simulink model "SD2231_Lab1_2024_PIDController"  (R2023a)
settings: Solver=FixedStepAuto  StartTime=0.0  StopTime=inf  FixedStep=0.001  RelTol=1e-3  EnableMultiTasking=on
values from neighbouring files (symbols this model uses):
  K_brake = K_brake(3)    [initial_student.m]    (also in initial_student_final.m)
  K_em = K_em(3)    [initial_student.m]    (also in initial_student_final.m)
undefined symbols (not defined in the file or in its folder): DiscIntNeverNeededParam, Veh
libraries: CarMaker4SL x37, SignalEditorBlockLib x2, autolibmappedmotor x2
(part 1 of 3)
settings Model: ExtModeTrigMode=oneshot  Creator=cs  LastModifiedBy=Student
settings SolverCC: AlgebraicLoopSolver=TrustRegion
settings DataIOCC: SaveFormat=Array  SignalLoggingSaveFormat=ModelDataLogs  ReturnWorkspaceOutputs=off  SignalLoggingName=sigsOut
settings OptimizationCC: BooleanDataType=off  OptimizeBlockIOStorage=off  BufferReuse=off  GlobalBufferReuse=off  ExpressionFolding=off  ExpressionDepthLimit=2147483647  LocalBlockOutputs=off  InitFltsAndDblsToZero=on  LifeSpan=inf  OptimizeDataStoreBuffers=off  BusAssignmentInplaceUpdate=off
settings DebuggingCC: SaveWithParameterizedLinksMsg=none  UnderspecifiedInitializationDetection=Classic  MergeDetectMultiDrivingBlocksExec=none  SignalResolutionControl=TryResolveAllWithWarning  MultiTaskDSMMsg=warning  MultiTaskCondExecSysMsg=none  FcnCallInpInsideContextMsg=warning  UnconnectedInputMsg=warning  UnconnectedOutputMsg=warning  UnconnectedLineMsg=warning  StateNameClashWarn=warning  SFUnexpectedBacktrackingDiag=warning  SFNoUnconditionalDefaultTransitionDiag=warning  ArithmeticOperatorsInVariantConditions=warning
settings HardwareCC: ProdBitPerPointer=32  ProdBitPerSizeT=32  ProdBitPerPtrDiffT=32  ProdLargestAtomicFloat=None  ProdIntDivRoundTo=Undefined  ProdEndianess=Unspecified  ProdWordSize=32  ProdHWDeviceType=32-bit Generic  TargetUnknown=on
settings ModelReferenceCC: EnableRefExpFcnMdlSchedulingChecks=on  PropagateSignalLabelsOutOfModel=off
settings SFSimCC: SimUseLocalCustomCode=off  CustomCodeUndefinedFunction=UseInterfaceOnly
settings RTWCC: SystemTargetFile=grt_malloc.tlc  TemplateMakefile=grt_malloc_default_tmf  RTWUseLocalCustomCode=off
settings CodeAppCC: MaxIdLength=63  StateflowObjectComments=on
settings GRTTargetCC: TargetFcnLib=ansi_tfl_tmw.mat  TargetLangStandard=C89/C90 (ANSI)  CombineOutputUpdateFcns=off  GRTInterface=on  UseMalloc=on  ExtModeMexFile=noextcomm
settings ConfigComp: CovMetricSettings=dw  CovSaveCumulativeToWorkspaceVar=on  CovSaveSingleToWorkspaceVar=on  CovExternalEMLEnable=off

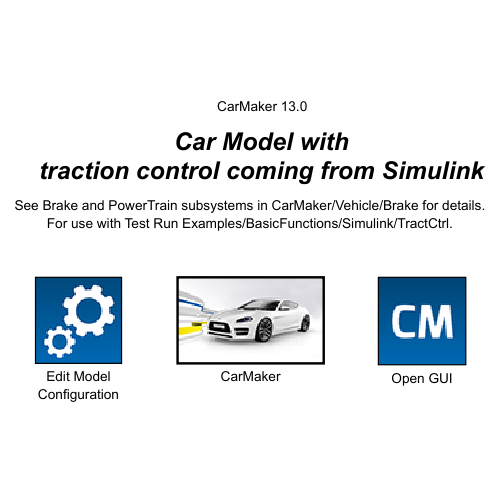
[thumbnail: Simulink's stored preview of the top-level diagram]
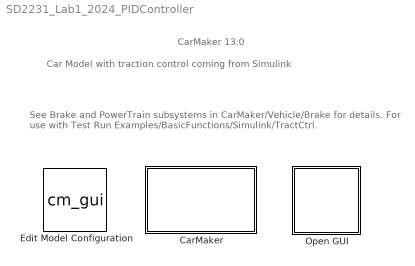
== system SD2231_Lab1_2024_PIDController ==
  note: Car Model with
      | traction control coming from Simulink
  note: See Brake and PowerTrain subsystems in CarMaker/Vehicle/Brake for details.
      | For use with Test Run Examples/BasicFunctions/Simulink/TractCtrl.
  note: CarMaker 13.0
  CarMaker : Subsystem  TreatAsAtomicUnit=on
      mask Display: image(imread('CarMakerSys.png'));
  Edit Model Configuration : S-Function  FunctionName=cm_gui  SFunctionDeploymentMode=off  EnableBusSupport=off
      settings: OpenFcn=cmmodelconf('edit');
      mask Display: image(imread('ModelConfig.png'));
  Open GUI : Subsystem  LoadFcn=if ~length(which('cmself')), cmenv; end
      settings: OpenFcn=cmblockmagic('gui_fix_display'); CM_Simulink
      mask Display: image(imread('CarMakerGUI.png'));

== system SD2231_Lab1_2024_PIDController/CarMaker ==
  Bus Creator : BusCreator  Inputs=6
  CM_FIRST : Subsystem
  CM_LAST : Subsystem
  CarMaker data : Subsystem
  DrivMan : Subsystem
  Ground : Ground
  IPG Vehicle : Subsystem
  Road friction : Subsystem
  Terminator : Terminator
  VehicleControl : Subsystem
  Your ABS Controller : Subsystem
  Your Traction Controller : Subsystem
  Your observer : Subsystem
  Your tyre force mapping : Subsystem
  wires:
  VehicleControl/2(Vhcl.Model.Source) -> IPG Vehicle/2(Vhcl.Model.Source)
  VehicleControl/7(VhclCtrl.PT) -> IPG Vehicle/7(VhclCtrl.PT)
  VehicleControl/6(VhclCtrl.Brake) -> IPG Vehicle/6(VhclCtrl.Brake)
  VehicleControl/5(Vhcl.Misc) -> IPG Vehicle/5(Vhcl.Misc)
  VehicleControl/4(Vhcl.Wheel.In) -> IPG Vehicle/4(Vhcl.Wheel.In)
  VehicleControl/3(VhclCtrl.Steering) -> IPG Vehicle/3(VhclCtrl.Steering)
  VehicleControl/1(Sync_Out) -> IPG Vehicle/1(Sync_In)
  IPG Vehicle/1(Sync_Out) -> CM_LAST/1(Sync_In)
  Ground/1 -> CM_FIRST/1(Sync_In)
  CM_LAST/1(Sync_Out) -> Terminator/1
  CM_FIRST/1(Sync_Out) -> DrivMan/1(Sync_In)
  CM_FIRST/2(Env.Misc) -> DrivMan/2(Env.Misc)
  DrivMan/1(Sync_Out) -> VehicleControl/1(Sync_In)
  DrivMan/2(DrivMan.Out) -> VehicleControl/2(DrivMan.In)
  Your ABS Controller/4(RRBrakeAdjust) -> Bus Creator/6
  Your observer/1(CarMaker bus data out) -> Your Traction Controller/1(CarMaker bus data), Your ABS Controller/1(CarMaker bus data)
  Your Traction Controller/2(RR TrqReqSignal (0-1)) -> Bus Creator/2
  Bus Creator/1 -> IPG Vehicle/8(SD2231.data)
  Your ABS Controller/2(FRBrakeAdjust) -> Bus Creator/4
  Your ABS Controller/1(FLBrakeAdjust) -> Bus Creator/3
  Your ABS Controller/3(RLBrakeAdjust) -> Bus Creator/5
  CarMaker data/1(CarMaker bus data) -> Your observer/1(CarMaker bus data)
  Your observer/2(Tyre slip bus data out) -> Your Traction Controller/2(Tyre slip bus data), Your tyre force mapping/1(Tyre slip bus data out), Your ABS Controller/2(Tyre slip bus data)
  Your Traction Controller/1(LR TrqReqSignal (0-1)) -> Bus Creator/1

== system SD2231_Lab1_2024_PIDController/Open GUI ==
  S-Function : S-Function  FunctionName=cm_gui  SFunctionDeploymentMode=off  EnableBusSupport=off

== system SD2231_Lab1_2024_PIDController/CarMaker/CM_FIRST ==
  Sync_In : Inport
  BusCreator1 : BusCreator  Inputs=8
  BusCreator2 : BusCreator  Inputs=6
  Demux1 : Demux  Outputs=14
      settings: DisplayOption=none
  Environment : S-Function  FunctionName=CM_Sfun  Parameters='Environment'  SFunctionDeploymentMode=off  EnableBusSupport=off
  IoIn : S-Function  FunctionName=CM_Sfun  Parameters='IoIn'  SFunctionDeploymentMode=off  EnableBusSupport=off
  Terminator : Terminator
  Sync_Out : Outport  VectorParamsAs1DForOutWhenUnconnected=off
  Env.Misc : Outport  Port=2  VectorParamsAs1DForOutWhenUnconnected=off
  wires:
  BusCreator2/1 -> Terminator/1  "IF Environment (in)"
  BusCreator1/1 -> Env.Misc/1
  Demux1/14 -> BusCreator2/6  "Env sRoad"
  Demux1/13 -> BusCreator2/5  "Env PoI_GCS Elev"
  Demux1/12 -> BusCreator2/4  "Env PoI_GCS Lat"
  Demux1/11 -> BusCreator2/3  "Env PoI_GCS Long"
  Demux1/10 -> BusCreator2/2  "Env Time"
  Demux1/9 -> BusCreator2/1  "Env yDay"
  Demux1/8 -> BusCreator1/8  "Env WindVel_tot z"
  Demux1/7 -> BusCreator1/7  "Env WindVel_tot y"
  Demux1/6 -> BusCreator1/6  "Env WindVel_tot x"
  Demux1/5 -> BusCreator1/5  "Env SolarRadiation"
  Demux1/4 -> BusCreator1/4  "Env AirHumidity"
  Demux1/3 -> BusCreator1/3  "Env AirPressure"
  Demux1/2 -> BusCreator1/2  "Env AirDensity"
  Demux1/1 -> BusCreator1/1  "Env Temperature"
  Environment/2 -> Demux1/1
  Environment/1 -> Sync_Out/1
  IoIn/1 -> Environment/1
  Sync_In/1 -> IoIn/1

== system SD2231_Lab1_2024_PIDController/CarMaker/CM_LAST ==
  Sync_In : Inport
  CM_User : S-Function  FunctionName=CM_Sfun  Parameters='CM_User'  SFunctionDeploymentMode=off  EnableBusSupport=off
  IoOut : S-Function  FunctionName=CM_Sfun  Parameters='IoOut'  SFunctionDeploymentMode=off  EnableBusSupport=off
  Sync_Out : Outport  VectorParamsAs1DForOutWhenUnconnected=off
  wires:
  IoOut/1 -> Sync_Out/1
  CM_User/1 -> IoOut/1
  Sync_In/1 -> CM_User/1

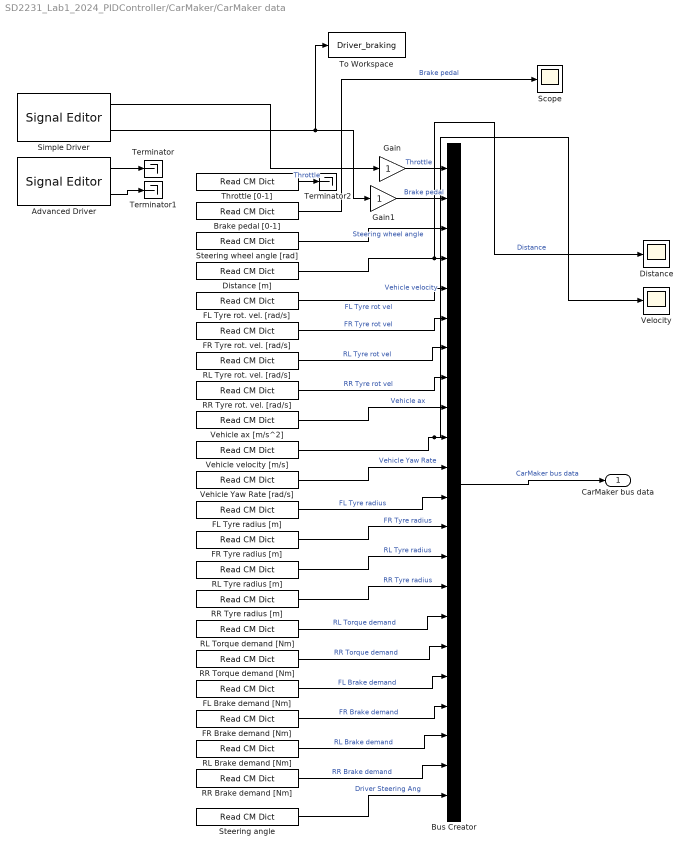
== system SD2231_Lab1_2024_PIDController/CarMaker/CarMaker data ==
  Advanced Driver : SignalEditorBlockLib/Signal Editor  FileName=DriverGas_Advanced.mat  ActiveScenario=Scenario  ActiveSignal=Brake  IsBus=off  OutputBusObjectStr=Bus: BusObject  SampleTime=0  ZeroCross=off  OutputAfterFinalValue=Holding final value  Unit=inherit  PreserveSignalName=on  ApplySigPropsToAllScenarios=off
  Brake pedal [0-1] : CarMaker4SL/Read CM Dict  xname=Driver.Brake  xsync=off  xstime=Continuous
  Bus Creator : BusCreator  Inputs=22
  Distance : Scope
  Distance [m] : CarMaker4SL/Read CM Dict  xname=Vhcl.Distance  xsync=off  xstime=Continuous
  FL Brake demand [Nm] : CarMaker4SL/Read CM Dict  xname=Vhcl.FL.Trq_Brake  xsync=off  xstime=Continuous
  FL Tyre radius [m] : CarMaker4SL/Read CM Dict  xname=Car.WFL.Radius  xsync=off  xstime=Continuous
  FL Tyre rot. vel. [rad/s] : CarMaker4SL/Read CM Dict  xname=Car.WheelSpd_FL  xsync=off  xstime=Continuous
  FR Brake demand [Nm] : CarMaker4SL/Read CM Dict  xname=Vhcl.FR.Trq_Brake  xsync=off  xstime=Continuous
  FR Tyre radius [m] : CarMaker4SL/Read CM Dict  xname=Car.WFR.Radius  xsync=off  xstime=Continuous
  FR Tyre rot. vel. [rad/s] : CarMaker4SL/Read CM Dict  xname=Car.WheelSpd_FR  xsync=off  xstime=Continuous
  Gain : Gain
  Gain1 : Gain
  RL Brake demand [Nm] : CarMaker4SL/Read CM Dict  xname=Vhcl.RL.Trq_Brake  xsync=off  xstime=Continuous
  RL Torque demand [Nm] : CarMaker4SL/Read CM Dict  xname=Vhcl.RL.Trq_T2W  xsync=off  xstime=Continuous
  RL Tyre radius [m] : CarMaker4SL/Read CM Dict  xname=Car.WRL.Radius  xsync=off  xstime=Continuous
  RL Tyre rot. vel. [rad/s] : CarMaker4SL/Read CM Dict  xname=Car.WheelSpd_RL  xsync=off  xstime=Continuous
  RR Brake demand [Nm] : CarMaker4SL/Read CM Dict  xname=Vhcl.RR.Trq_Brake  xsync=off  xstime=Continuous
  RR Torque demand [Nm] : CarMaker4SL/Read CM Dict  xname=Vhcl.RR.Trq_T2W  xsync=off  xstime=Continuous
  RR Tyre radius [m] : CarMaker4SL/Read CM Dict  xname=Car.WRR.Radius  xsync=off  xstime=Continuous
  RR Tyre rot. vel. [rad/s] : CarMaker4SL/Read CM Dict  xname=Car.WheelSpd_RR  xsync=off  xstime=Continuous
  Scope : Scope
  Simple Driver : SignalEditorBlockLib/Signal Editor  FileName=DriverGas.mat  ActiveScenario=Scenario  ActiveSignal=Brake  IsBus=off  OutputBusObjectStr=Bus: BusObject  SampleTime=0  ZeroCross=off  OutputAfterFinalValue=Holding final value  Unit=inherit  PreserveSignalName=on  ApplySigPropsToAllScenarios=off
  Steering angle : CarMaker4SL/Read CM Dict  xname=Driver.Steer.Ang  xsync=off  xstime=Continuous
  Steering wheel angle [rad] : CarMaker4SL/Read CM Dict  xname=Driver.Steer.Ang  xsync=off  xstime=Continuous
  Terminator : Terminator
  Terminator1 : Terminator
  Terminator2 : Terminator
  Throttle [0-1] : CarMaker4SL/Read CM Dict  xname=Driver.Gas  xsync=off  xstime=Continuous
  To Workspace : ToWorkspace  VariableName=Driver_braking  SaveFormat=Timeseries  SampleTime=-1
  Vehicle Yaw Rate [rad/s] : CarMaker4SL/Read CM Dict  xname=Car.YawRate  xsync=off  xstime=Continuous
  Vehicle ax [m/s^2] : CarMaker4SL/Read CM Dict  xname=Car.ax  xsync=off  xstime=Continuous
  Vehicle velocity [m/s] : CarMaker4SL/Read CM Dict  xname=Car.v  xsync=off  xstime=Continuous
  Velocity : Scope
  CarMaker bus data : Outport  VectorParamsAs1DForOutWhenUnconnected=off
  wires:
  RR Tyre rot. vel. [rad/s]/1 -> Bus Creator/8  "RR Tyre rot vel"
  RL Tyre rot. vel. [rad/s]/1 -> Bus Creator/7  "RL Tyre rot vel"
  Distance [m]/1 -> Distance/1, Bus Creator/4  "Distance"
  FR Tyre rot. vel. [rad/s]/1 -> Bus Creator/6  "FR Tyre rot vel"
  Brake pedal [0-1]/1 -> Scope/1  "Brake pedal"
  Vehicle ax [m/s^2]/1 -> Bus Creator/9  "Vehicle ax"
  Steering wheel angle [rad]/1 -> Bus Creator/3  "Steering wheel angle"
  Throttle [0-1]/1 -> Terminator2/1  "Throttle"
  Vehicle velocity [m/s]/1 -> Velocity/1, Bus Creator/10  "Vehicle velocity"
  FL Tyre rot. vel. [rad/s]/1 -> Bus Creator/5  "FL Tyre rot vel"
  Vehicle Yaw Rate [rad/s]/1 -> Bus Creator/11  "Vehicle Yaw Rate"
  FL Tyre radius [m]/1 -> Bus Creator/12  "FL Tyre radius"
  FR Tyre radius [m]/1 -> Bus Creator/13  "FR Tyre radius"
  RL Tyre radius [m]/1 -> Bus Creator/14  "RL Tyre radius"
  RR Tyre radius [m]/1 -> Bus Creator/15  "RR Tyre radius"
  Bus Creator/1 -> CarMaker bus data/1  "CarMaker bus data"
  RL Torque demand [Nm]/1 -> Bus Creator/16  "RL Torque demand"
  RR Torque demand [Nm]/1 -> Bus Creator/17  "RR Torque demand"
  FL Brake demand [Nm]/1 -> Bus Creator/18  "FL Brake demand"
  FR Brake demand [Nm]/1 -> Bus Creator/19  "FR Brake demand"
  RL Brake demand [Nm]/1 -> Bus Creator/20  "RL Brake demand"
  RR Brake demand [Nm]/1 -> Bus Creator/21  "RR Brake demand"
  Gain/1 -> Bus Creator/1  "Throttle"
  Gain1/1 -> Bus Creator/2  "Brake pedal"
  Steering angle/1 -> Bus Creator/22  "Driver Steering Ang"
  Simple Driver/1 -> Gain/1
  Advanced Driver/1 -> Terminator/1
  Simple Driver/2 -> To Workspace/1, Gain1/1
  Advanced Driver/2 -> Terminator1/1

== system SD2231_Lab1_2024_PIDController/CarMaker/DrivMan ==
  note: There's rarely a reason to override DrivMan signals.
      | Use the VehicleControl interface for this purpose.
  Sync_In : Inport
  Env.Misc : Inport  Port=2
  BusCreator : BusCreator  Inputs=20
  Demux : Demux  Outputs=20
      settings: DisplayOption=none
  DrivMan : S-Function  FunctionName=CM_Sfun  Parameters='DrivMan'  SFunctionDeploymentMode=off  EnableBusSupport=off
  Sync_Out : Outport  VectorParamsAs1DForOutWhenUnconnected=off
  DrivMan.Out : Outport  Port=2  VectorParamsAs1DForOutWhenUnconnected=off
  wires:
  Demux/8 -> BusCreator/8  "DrivMan SelectorCtrl"
  Demux/7 -> BusCreator/7  "DrivMan UserSignal4"
  Demux/6 -> BusCreator/6  "DrivMan UserSignal3"
  Demux/5 -> BusCreator/5  "DrivMan UserSignal2"
  Demux/4 -> BusCreator/4  "DrivMan UserSignal1"
  Demux/3 -> BusCreator/3  "DrivMan UserSignal0"
  Demux/2 -> BusCreator/2  "DrivMan Key"
  Demux/1 -> BusCreator/1  "DrivMan SST"
  Env.Misc/1 -> DrivMan/2
  Sync_In/1 -> DrivMan/1
  DrivMan/1 -> Sync_Out/1
  BusCreator/1 -> DrivMan.Out/1
  DrivMan/2 -> Demux/1
  Demux/9 -> BusCreator/9  "DrivMan DigitalSelectorCtrl0"
  Demux/10 -> BusCreator/10  "DrivMan DigitalSelectorCtrl1"
  Demux/11 -> BusCreator/11  "DrivMan DigitalSelectorCtrl2"
  Demux/20 -> BusCreator/20  "DrivMan Steering Trq"
  Demux/19 -> BusCreator/19  "DrivMan Steering AngAcc"
  Demux/18 -> BusCreator/18  "DrivMan Steering AngVel"
  Demux/17 -> BusCreator/17  "DrivMan Steering Ang"
  Demux/16 -> BusCreator/16  "DrivMan Gas"
  Demux/15 -> BusCreator/15  "DrivMan Clutch"
  Demux/14 -> BusCreator/14  "DrivMan BrakePark"
  Demux/13 -> BusCreator/13  "DrivMan Brake"
  Demux/12 -> BusCreator/12  "DrivMan GearNo"

== system SD2231_Lab1_2024_PIDController/CarMaker/IPG Vehicle ==
  Sync_In : Inport
  Vhcl.Model.Source : Inport  Port=2
  VhclCtrl.Steering : Inport  Port=3
  Vhcl.Wheel.In : Inport  Port=4
  Vhcl.Misc : Inport  Port=5
  VhclCtrl.Brake : Inport  Port=6
  VhclCtrl.PT : Inport  Port=7
  SD2231.data : Inport  Port=8
  Brake : Subsystem
  CarAndTrailer : Subsystem
  PowerTrain : Subsystem
  Stop Simulation : Stop
  VehicleSource_BuiltIn : Subsystem  mask(Compare To Constant){relop=~=, const=1, OutDataTypeStr=boolean, ZeroCross=off}
      mask prompts: relop "Simulink:masks:Operator_MP"; const "Simulink:masks:ConstantValue_MP"; OutDataTypeStr "Simulink:masks:OutputDataType_MP"; ZeroCross "Simulink:masks:EnableZerocrossingDetection_MP"
      mask help: Simulink:masks:CompareToConstant_MD
      mask init:
      | blkName = gcb;
      | 
      | if strcmp(get_param(gcbh,'OutDataTypeStr'),'boolean')
      | 	setValue = 'boolean';
      | else
      | 	setValue = 'fixdt(0, 8)';
      | end
      | 
      | set_param([blkName,'/Compare'],'relop',relop, ...
      | 	'OutDataTypeStr', setValue, 'ZeroCross', ZeroCross);
      | 
      | str = [relop,' C']; %default
      | 
      | const_str = get_param(blkName, 'const');
      | 
      | if isempty(strfind(const_str, ' ')) && isempty(strfind(const_str, ','))
      |     % scalar or single expression
      |     if isempty(str2num(const_str))
      |         %expression
      |         str = [relop, ' ', const_str];
      |     elseif length(const) == 1
      |         str = [relop,' ',num2str(double(const))];
      |     end
      | end
      mask TypeOptions relop: == | ~= | < | <= | >= | >
      mask TypeOptions OutDataTypeStr: Simulink:masks:uint8 | Simulink:masks:boolean
      mask Callback ZeroCross: sl('zeroCrossEnable', gcbh);
      mask Display: disp(str)
  Sync_Out : Outport  VectorParamsAs1DForOutWhenUnconnected=off
  wires:
  VhclCtrl.PT/1 -> PowerTrain/3(VhclCtrl.PT)
  Brake/1(Sync_Out) -> PowerTrain/1(Sync_In)
  CarAndTrailer/1(Sync_Out) -> Brake/1(Sync_In)
  CarAndTrailer/2(Brake.IF.In) -> Brake/2(Brake.IF.In)
  VhclCtrl.Brake/1 -> Brake/3(VhclCtrl.Brake)
  PowerTrain/1(Sync_Out) -> Sync_Out/1
  Vhcl.Misc/1 -> CarAndTrailer/4(Vhcl.Misc)
  Vhcl.Wheel.In/1 -> CarAndTrailer/3(Vhcl.Wheel.In)
  VhclCtrl.Steering/1 -> CarAndTrailer/2(VhclCtrl.Steering)
  Sync_In/1 -> CarAndTrailer/1(Sync_In)
  Vhcl.Model.Source/1 -> VehicleSource_BuiltIn/1(u)
  VehicleSource_BuiltIn/1(y) -> Stop Simulation/1
  Brake/2(Vhcl.Wheel.PT) -> PowerTrain/2(Vhcl.Wheel.PT)
  SD2231.data/1 -> PowerTrain/6(SD2232.data), Brake/4(SD2231.Data)
  CarAndTrailer/3(Car.Trq_T2W) -> PowerTrain/5(Car.TrqT2W)
  Brake/3(Brake.IF.Out) -> PowerTrain/4(Brake.IF.Out)

== system SD2231_Lab1_2024_PIDController/CarMaker/Road friction ==
  Constant : Constant  Value=Veh.mu
  Write CM Dict : CarMaker4SL/Write CM Dict  xname=Car.muRoadFL  xsync=off
  Write CM Dict1 : CarMaker4SL/Write CM Dict  xname=Car.muRoadFR  xsync=off
  Write CM Dict2 : CarMaker4SL/Write CM Dict  xname=Car.muRoadRL  xsync=off
  Write CM Dict3 : CarMaker4SL/Write CM Dict  xname=Car.muRoadRR  xsync=off
  wires:
  Constant/1 -> Write CM Dict1/1, Write CM Dict/1, Write CM Dict3/1, Write CM Dict2/1

== system SD2231_Lab1_2024_PIDController/CarMaker/VehicleControl ==
  note: <Your model here>
  note: When implementing a vehicle control model,
      | be sure to add '-disablevehiclecontrol' to the command line arguments
      | in the CarMaker Model Configuration block.
      | Otherwise your model will possibly not see the original DrivMan signals
      | on its inputs, but those of a currently activated C-coded vehicle control model instead.
  Sync_In : Inport
  DrivMan.In : Inport  Port=2
  Bus Creator2 : BusCreator  Inputs=2
  CreateBus Vhcl.Misc : Subsystem
  CreateBus Vhcl.Wheel.In : Subsystem
  CreateBus VhclCtrl : Subsystem
  CreateBus VhclCtrl.PT : Subsystem
  CreateBus VhclCtrl.Steering : Subsystem
  Demux2 : Demux  Outputs=2
      settings: DisplayOption=none
  VehicleControl : S-Function  FunctionName=CM_Sfun  Parameters='VehicleControl'  SFunctionDeploymentMode=off  EnableBusSupport=off
  VehicleControlUpd : S-Function  FunctionName=CM_Sfun  Parameters='VehicleControlUpd'  SFunctionDeploymentMode=off  EnableBusSupport=off
  Sync_Out : Outport  VectorParamsAs1DForOutWhenUnconnected=off
  Vhcl.Model.Source : Outport  Port=2  VectorParamsAs1DForOutWhenUnconnected=off
  VhclCtrl.Steering : Outport  Port=3  VectorParamsAs1DForOutWhenUnconnected=off
  Vhcl.Wheel.In : Outport  Port=4  VectorParamsAs1DForOutWhenUnconnected=off
  Vhcl.Misc : Outport  Port=5  VectorParamsAs1DForOutWhenUnconnected=off
  VhclCtrl.Brake : Outport  Port=6  VectorParamsAs1DForOutWhenUnconnected=off
  VhclCtrl.PT : Outport  Port=7  VectorParamsAs1DForOutWhenUnconnected=off
  wires:
  CreateBus VhclCtrl/1(Out) -> VehicleControlUpd/2
  VehicleControl/2 -> CreateBus VhclCtrl/1(In)
  VehicleControlUpd/2 -> Vhcl.Model.Source/1
  VehicleControlUpd/4 -> CreateBus Vhcl.Wheel.In/1(In1)
  VehicleControlUpd/5 -> CreateBus Vhcl.Misc/1(In1)
  VehicleControlUpd/6 -> Demux2/1
  VehicleControlUpd/7 -> CreateBus VhclCtrl.PT/1(In1)
  VehicleControlUpd/3 -> CreateBus VhclCtrl.Steering/1(In1)
  CreateBus Vhcl.Misc/1(Out1) -> Vhcl.Misc/1
  CreateBus Vhcl.Wheel.In/1(Out1) -> Vhcl.Wheel.In/1
  DrivMan.In/1 -> VehicleControl/2
  VehicleControl/1 -> VehicleControlUpd/1
  Sync_In/1 -> VehicleControl/1
  CreateBus VhclCtrl.PT/1(Out1) -> VhclCtrl.PT/1
  Bus Creator2/1 -> VhclCtrl.Brake/1
  CreateBus VhclCtrl.Steering/1(Out1) -> VhclCtrl.Steering/1
  VehicleControlUpd/1 -> Sync_Out/1
  Demux2/2 -> Bus Creator2/2  "VhclCtrl BrakePark"
  Demux2/1 -> Bus Creator2/1  "VhclCtrl Brake"

== system SD2231_Lab1_2024_PIDController/CarMaker/Your ABS Controller ==
  CarMaker bus data : Inport
  Tyre slip bus data : Inport  Port=2
  Bus Selector : BusSelector  OutputSignals=Brake pedal,Vehicle velocity
  Bus Selector1 : BusSelector  OutputSignals=FL Braking Slip,RL Braking Slip
  Gain{,1..3} (4 alike) : Gain
  P Controller : Subsystem
  PD Controller : Subsystem
  PI Controller : Subsystem
  PID Controller : Subsystem
  Terminator{,1..5} (6 alike) : Terminator
  FLBrakeAdjust : Outport  VectorParamsAs1DForOutWhenUnconnected=off
  FRBrakeAdjust : Outport  Port=2  VectorParamsAs1DForOutWhenUnconnected=off
  RLBrakeAdjust : Outport  Port=3  VectorParamsAs1DForOutWhenUnconnected=off
  RRBrakeAdjust : Outport  Port=4  VectorParamsAs1DForOutWhenUnconnected=off
  wires:
  Gain1/1 -> RLBrakeAdjust/1  "RLBrakeAdjust"
  Bus Selector/1 -> PI Controller/3(<Brake pedal>), PID Controller/3(<Brake pedal>), PD Controller/3(<Brake pedal>), P Controller/3(<Brake pedal>)  "<Brake pedal>"
  CarMaker bus data/1 -> Bus Selector/1
  Gain/1 -> FRBrakeAdjust/1  "FRBrakeAdjust"
  Gain2/1 -> RRBrakeAdjust/1  "RRBrakeAdjust"
  Gain3/1 -> FLBrakeAdjust/1  "FLBrakeAdjust"
  Tyre slip bus data/1 -> Bus Selector1/1
  Bus Selector1/1 -> PID Controller/1(<FL Braking Slip>), PD Controller/1(<FL Braking Slip>), PI Controller/1(<FL Braking Slip>), P Controller/1(<FL Braking Slip>)  "<FL Braking Slip>"
  Bus Selector1/2 -> P Controller/2(<RL Braking Slip>), PI Controller/2(<RL Braking Slip>), PD Controller/2(<RL Braking Slip>), PID Controller/2(<RL Braking Slip>)  "<RL Braking Slip>"
  Bus Selector/2 -> PID Controller/4(Vehicle_Velocity), PD Controller/4(Vehicle_Velocity), PI Controller/4(Vehicle_Velocity), P Controller/4(Vehicle_Velocity)  "<Vehicle velocity>"
  P Controller/1(Front_Braking) -> Terminator2/1
  P Controller/2(Rear_Braking) -> Terminator5/1
  PI Controller/2(Rear_Braking) -> Terminator3/1
  PI Controller/1(Front_Braking) -> Terminator1/1
  PD Controller/2(Rear_Braking) -> Terminator4/1
  PD Controller/1(Front_Braking) -> Terminator/1
  PID Controller/1(Front_Braking) -> Gain/1, Gain3/1
  PID Controller/2(Rear_Braking) -> Gain2/1, Gain1/1

== system SD2231_Lab1_2024_PIDController/CarMaker/Your Traction Controller ==
  note: Signal out 1 should have name "LRTrqAdjust"
      | Signal out 2 should have name "RRTrqAdjust"
  CarMaker bus data : Inport
  Tyre slip bus data : Inport  Port=2
  Bus Selector : BusSelector  OutputSignals=Throttle
  Bus Selector1 : BusSelector  OutputSignals=RL Tractive Slip
  Gain : Gain
  Gain1 : Gain
  Terminator : Terminator
  LR TrqReqSignal (0-1) : Outport  VectorParamsAs1DForOutWhenUnconnected=off
  RR TrqReqSignal (0-1) : Outport  Port=2  VectorParamsAs1DForOutWhenUnconnected=off
  wires:
  Tyre slip bus data/1 -> Bus Selector1/1  "RRTrqAdjust"
  CarMaker bus data/1 -> Bus Selector/1
  Bus Selector/1 -> Gain1/1, Gain/1  "<Throttle>"
  Bus Selector1/1 -> Terminator/1  "<RL Tractive Slip>"
  Gain/1 -> LR TrqReqSignal (0-1)/1  "LRTrqAdjust"
  Gain1/1 -> RR TrqReqSignal (0-1)/1  "RRTrqAdjust"

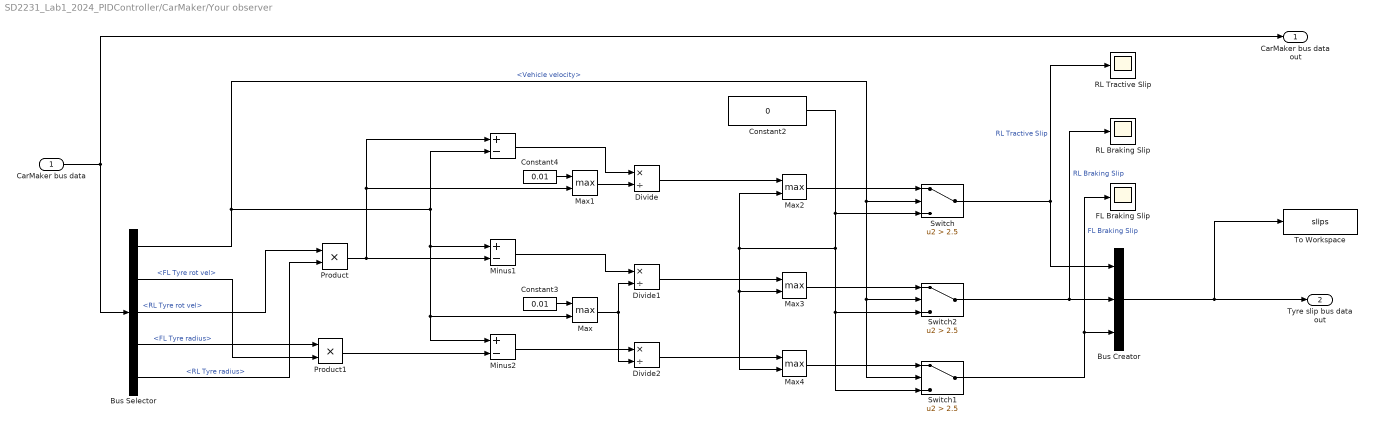
== system SD2231_Lab1_2024_PIDController/CarMaker/Your observer ==
  CarMaker bus data : Inport
  " " : Sum  Inputs=+-
  Bus Creator : BusCreator  Inputs=3
  Bus Selector : BusSelector  OutputSignals=Vehicle velocity,FL Tyre rot vel,RL Tyre rot vel,FL Tyre radius,RL Tyre radius
  Constant2 : Constant  Value=0
  Constant3 : Constant  Value=0.01
  Constant4 : Constant  Value=0.01
  Divide : Product  Inputs=*/
  Divide1 : Product  Inputs=*/
  Divide2 : Product  Inputs=*/
  FL Braking Slip : Scope
  Max{,1..4} (5 alike) : MinMax  Function=max  Inputs=2
  Minus1 : Sum  Inputs=+-
  Minus2 : Sum  Inputs=+-
  Product : Product
  Product1 : Product
  RL Braking Slip : Scope
  RL Tractive Slip : Scope
  Switch : Switch  Criteria=u2 > Threshold  Threshold=2.5  SaturateOnIntegerOverflow=off  InputSameDT=off
  Switch1 : Switch  Criteria=u2 > Threshold  Threshold=2.5  SaturateOnIntegerOverflow=off  InputSameDT=off
  Switch2 : Switch  Criteria=u2 > Threshold  Threshold=2.5  SaturateOnIntegerOverflow=off  InputSameDT=off
  To Workspace : ToWorkspace  VariableName=slips  SaveFormat=Timeseries  SampleTime=-1
  CarMaker bus data out : Outport  VectorParamsAs1DForOutWhenUnconnected=off
  Tyre slip bus data out : Outport  Port=2  VectorParamsAs1DForOutWhenUnconnected=off
  wires:
  CarMaker bus data/1 -> Bus Selector/1, CarMaker bus data out/1
  Bus Creator/1 -> To Workspace/1, Tyre slip bus data out/1
  Divide/1 -> Max2/1
  " "/1 -> Divide/1
  Bus Selector/5 -> Product/2  "<RL Tyre radius>"
  Minus1/1 -> Divide1/1
  Divide1/1 -> Max3/1
  Product1/1 -> Minus2/2
  Minus2/1 -> Divide2/1
  Divide2/1 -> Max4/1
  Bus Selector/4 -> Product1/1  "<FL Tyre radius>"
  Bus Selector/3 -> Product/1  "<RL Tyre rot vel>"
  Bus Selector/2 -> Product1/2  "<FL Tyre rot vel>"
  Bus Selector/1 -> Switch/2, Switch1/2, Switch2/2, Max/2, Minus2/1, Minus1/1, " "/2  "<Vehicle velocity>"
  Constant3/1 -> Max/1
  Product/1 -> Minus1/2, " "/1, Max1/2
  Max/1 -> Divide1/2, Divide2/2
  Max1/1 -> Divide/2
  Constant2/1 -> Switch1/3, Switch2/3, Max2/2, Max3/2, Max4/2, Switch/3
  Switch/1 -> Bus Creator/1, RL Tractive Slip/1  "RL Tractive Slip"
  Max2/1 -> Switch/1
  Max3/1 -> Switch2/1
  Switch2/1 -> Bus Creator/2, RL Braking Slip/1  "RL Braking Slip"
  Max4/1 -> Switch1/1
  Switch1/1 -> Bus Creator/3, FL Braking Slip/1  "FL Braking Slip"
  Constant4/1 -> Max1/1

== system SD2231_Lab1_2024_PIDController/CarMaker/Your tyre force mapping ==
  note: Ad the rest of the data you need to
      | the workspace from your model
  Tyre slip bus data out : Inport
  Bus Selector : BusSelector  OutputSignals=RL Tractive Slip,RL Braking Slip
  Read CM Dict : CarMaker4SL/Read CM Dict  xname=Car.FxFL  xsync=off  xstime=Continuous
  Read CM Dict1 : CarMaker4SL/Read CM Dict  xname=Car.ax  xsync=off  xstime=Continuous
  Read CM Dict2 : CarMaker4SL/Read CM Dict  xname=Car.FzFL  xsync=off  xstime=Continuous
  Read CM Dict3 : CarMaker4SL/Read CM Dict  xname=Car.FzRL  xsync=off  xstime=Continuous
  Read CM Dict4 : CarMaker4SL/Read CM Dict  xname=Car.FxRL  xsync=off  xstime=Continuous
  Terminator : Terminator
  Terminator1 : Terminator
  To Workspace : ToWorkspace  VariableName=ax  SampleTime=-1
  To Workspace1 : ToWorkspace  VariableName=FxFL  SaveFormat=Timeseries  SampleTime=-1
  To Workspace2 : ToWorkspace  VariableName=FzFL  SaveFormat=Timeseries  SampleTime=-1
  To Workspace3 : ToWorkspace  VariableName=FxRL  SaveFormat=Timeseries  SampleTime=-1
  To Workspace4 : ToWorkspace  VariableName=FzRL  SaveFormat=Timeseries  SampleTime=-1
  wires:
  Read CM Dict1/1 -> To Workspace/1
  Tyre slip bus data out/1 -> Bus Selector/1
  Bus Selector/1 -> Terminator/1  "<RL Tractive Slip>"
  Bus Selector/2 -> Terminator1/1  "<RL Braking Slip>"
  Read CM Dict/1 -> To Workspace1/1
  Read CM Dict2/1 -> To Workspace2/1
  Read CM Dict4/1 -> To Workspace3/1
  Read CM Dict3/1 -> To Workspace4/1

== system SD2231_Lab1_2024_PIDController/CarMaker/IPG Vehicle/Brake ==
  note: When replacing the entire braking system,
      | be sure to disable the IPG brake model by using the brake
      | model 'Model Manager off' in the vehicle GUI.
  Sync_In : Inport
  Brake.IF.In : Inport  Port=2
  VhclCtrl.Brake : Inport  Port=3
  SD2231.Data : Inport  Port=4
  Brake : S-Function  FunctionName=CM_Sfun  Parameters='Brake'  SFunctionDeploymentMode=off  EnableBusSupport=off
  BrakeUpd : S-Function  FunctionName=CM_Sfun  Parameters='BrakeUpd'  SFunctionDeploymentMode=off  EnableBusSupport=off
  BusCreator1 : BusCreator  Inputs=16
  CreateBus Vhcl.Wheel.PT : Subsystem
  Demux : Demux  Outputs=16
      settings: DisplayOption=none
  Terminator : Terminator
  UserDefinedBrakingSystem : Subsystem  TreatAsAtomicUnit=on
  Sync_Out : Outport  VectorParamsAs1DForOutWhenUnconnected=off
  Vhcl.Wheel.PT : Outport  Port=2  VectorParamsAs1DForOutWhenUnconnected=off
  Brake.IF.Out : Outport  Port=3  VectorParamsAs1DForOutWhenUnconnected=off
  wires:
  Demux/16 -> BusCreator1/16  "Brake IF Trq_DriveSrc_trg d3"
  Demux/15 -> BusCreator1/15  "Brake IF Trq_DriveSrc_trg d2"
  Demux/14 -> BusCreator1/14  "Brake IF Trq_DriveSrc_trg d1"
  Demux/13 -> BusCreator1/13  "Brake IF Trq_DriveSrc_trg d0"
  Demux/12 -> BusCreator1/12  "Brake IF Trq_Reg_trg RR"
  Demux/11 -> BusCreator1/11  "Brake IF Trq_Reg_trg RL"
  Demux/10 -> BusCreator1/10  "Brake IF Trq_Reg_trg FR"
  Demux/9 -> BusCreator1/9  "Brake IF Trq_Reg_trg FL"
  Demux/8 -> BusCreator1/8  "Brake IF Trq_PB RR"
  Demux/7 -> BusCreator1/7  "Brake IF Trq_PB RL"
  Demux/6 -> BusCreator1/6  "Brake IF Trq_PB FR"
  Demux/5 -> BusCreator1/5  "Brake IF Trq_PB FL"
  Demux/4 -> BusCreator1/4  "Brake IF Trq_WB RR"
  Demux/3 -> BusCreator1/3  "Brake IF Trq_WB RL"
  Brake/2 -> Terminator/1
  BusCreator1/1 -> Brake.IF.Out/1, BrakeUpd/2
  BrakeUpd/1 -> Sync_Out/1
  Brake/1 -> BrakeUpd/1  "Sync"
  Brake.IF.In/1 -> Brake/2
  VhclCtrl.Brake/1 -> Brake/3
  Sync_In/1 -> Brake/1
  BrakeUpd/2 -> CreateBus Vhcl.Wheel.PT/1(In)
  CreateBus Vhcl.Wheel.PT/1(Out) -> Vhcl.Wheel.PT/1
  UserDefinedBrakingSystem/1(Brake.IF.Out) -> Demux/1
  Demux/1 -> BusCreator1/1  "Brake IF Trq_WB FL"
  Demux/2 -> BusCreator1/2  "Brake IF Trq_WB FR"
  SD2231.Data/1 -> UserDefinedBrakingSystem/1(SD2231.Data)

== system SD2231_Lab1_2024_PIDController/CarMaker/IPG Vehicle/CarAndTrailer ==
  Sync_In : Inport
  VhclCtrl.Steering : Inport  Port=2
  Vhcl.Wheel.In : Inport  Port=3
  Vhcl.Misc : Inport  Port=4
  CarAndTrailerUpd : Subsystem
  Forces : Subsystem
  Ground : Ground
  Kinematics : Subsystem
  Kinetics : Subsystem
  Steering : Subsystem
  Terminator : Terminator
  Terminator1 : Terminator
  Trailer : Subsystem
  Sync_Out : Outport  VectorParamsAs1DForOutWhenUnconnected=off
  Brake.IF.In : Outport  Port=2  VectorParamsAs1DForOutWhenUnconnected=off
  Car.Trq_T2W : Outport  Port=3  VectorParamsAs1DForOutWhenUnconnected=off
  wires:
  Trailer/9(Car.Hitch.FrcTrq) -> CarAndTrailerUpd/9(Car.Hitch.FrcTrq)
  Trailer/8(Vhcl.Wheel.RR) -> CarAndTrailerUpd/8(Vhcl.Wheel.RR)
  Trailer/7(Vhcl.Wheel.RL) -> CarAndTrailerUpd/7(Vhcl.Wheel.RL)
  Trailer/6(Vhcl.Wheel.FR) -> CarAndTrailerUpd/6(Vhcl.Wheel.FR)
  Trailer/5(Vhcl.Wheel.FL) -> CarAndTrailerUpd/5(Vhcl.Wheel.FL)
  Trailer/4(Vhcl.PoI) -> CarAndTrailerUpd/4(Vhcl.PoI)
  Trailer/3(Vhcl.Motion) -> CarAndTrailerUpd/3(Vhcl.Motion)
  Trailer/2(Vhcl.Steering) -> CarAndTrailerUpd/2(Vhcl.Steering)
  Trailer/1(Sync_Out) -> CarAndTrailerUpd/1(Sync_In)
  CarAndTrailerUpd/2(Brake.IF.In) -> Brake.IF.In/1
  CarAndTrailerUpd/1(Sync_Out) -> Sync_Out/1
  Vhcl.Misc/1 -> Terminator1/1
  Vhcl.Wheel.In/1 -> Terminator/1
  Kinetics/6(WheelCarrier.Misc) -> Trailer/6(WheelCarrier.Misc)
  Kinetics/5(Car.Trq_T2W) -> Car.Trq_T2W/1, Trailer/5(Car.Trq_T2W)
  Steering/2(Steer.IF) -> Kinematics/2(Steer.IF)
  Kinetics/4(Car.Fr1) -> Trailer/4(Car.Fr1)
  Kinetics/3(Car.Hitch) -> Trailer/3(Car.Hitch)
  Kinetics/2(Trailer.Load) -> Trailer/2(Trailer.Load)
  VhclCtrl.Steering/1 -> Steering/2(VhclCtrl.Steering)
  Sync_In/1 -> Steering/1(Sync_In)
  Steering/1(Sync_Out) -> Kinematics/1(Sync_In)
  Kinetics/1(Sync_Out) -> Trailer/1(Sync_In)
  Ground/1 -> CarAndTrailerUpd/10(Vhcl.Fr1A)
  Forces/11(FStabi_ext) -> Kinetics/11(FStabi_ext)
  Forces/10(FDamp_ext) -> Kinetics/10(FDamp_ext)
  Forces/9(FSpring_ext) -> Kinetics/9(FSpring_ext)
  Forces/8(TireRR_Out) -> Kinetics/8(TireRR.Out)
  Forces/7(TireRL_Out) -> Kinetics/7(TireRL.Out)
  Forces/6(TireFR_Out) -> Kinetics/6(TireFR.Out)
  Forces/5(TireFL_Out) -> Kinetics/5(TireFL.Out)
  Forces/4(Car.Load) -> Kinetics/4(Car.Load)
  Forces/2(Car.Virtual) -> Kinetics/2(Car.Virtual)
  Kinematics/6(lSpring) -> Forces/6(lSpring)
  Kinematics/7(vDamp) -> Forces/7(vDamp)
  Forces/3(Car.Aero) -> Kinetics/3(Car.Aero)
  Forces/1(Sync_Out) -> Kinetics/1(Sync_In)
  Kinematics/5(TireRR_In) -> Forces/5(TireRR_In)
  Kinematics/4(TireRL_In) -> Forces/4(TireRL_In)
  Kinematics/3(TireFR_In) -> Forces/3(TireFR_In)
  Kinematics/2(TireFL_In) -> Forces/2(TireFL_In)
  Kinematics/1(Sync_Out) -> Forces/1(Sync_In)
  Kinematics/8(lStabi) -> Forces/8(lStabi)
  Forces/12(FBuf_ext) -> Kinetics/12(FBuf_ext)
  Kinematics/9(lBuf) -> Forces/9(lBuf)

== system SD2231_Lab1_2024_PIDController/CarMaker/IPG Vehicle/PowerTrain ==
  note: When replacing the entire powertrain,
      | be sure to disable the IPG powertrain model by using the powertrain
      | model 'Model Manager off' in the vehicle GUI.
  Sync_In : Inport
  Vhcl.Wheel.PT : Inport  Port=2
  VhclCtrl.PT : Inport  Port=3
  Brake.IF.Out : Inport  Port=4
  Car.TrqT2W : Inport  Port=5
  SD2232.data : Inport  Port=6
  BusCreator1 : BusCreator  Inputs=42
  Demux1 : Demux  Outputs=42
      settings: DisplayOption=none
  PowerTrain : S-Function  FunctionName=CM_Sfun  Parameters='PowerTrain'  SFunctionDeploymentMode=off  EnableBusSupport=off
  PowerTrainUpd : S-Function  FunctionName=CM_Sfun  Parameters='PowerTrainUpd'  SFunctionDeploymentMode=off  EnableBusSupport=off
  Terminator : Terminator
  User RearDriven PowerTrain : Subsystem
  Sync_Out : Outport  VectorParamsAs1DForOutWhenUnconnected=off
  wires:
  BusCreator1/1 -> PowerTrainUpd/2
  Demux1/42 -> BusCreator1/42  "PT IF WRR Trq_BrakeReg_max"
  Demux1/41 -> BusCreator1/41  "PT IF WRR Trq_BrakeReg"
  Demux1/40 -> BusCreator1/40  "PT IF WRR Trq_Supp2WC"
  Demux1/39 -> BusCreator1/39  "PT IF WRR Trq_Drive"
  Demux1/38 -> BusCreator1/38  "PT IF WRR Trq_B2W"
  Demux1/37 -> BusCreator1/37  "PT IF WRR rotv"
  Demux1/36 -> BusCreator1/36  "PT IF WRR rot"
  Demux1/35 -> BusCreator1/35  "PT IF WRL Trq_BrakeReg_max"
  Demux1/34 -> BusCreator1/34  "PT IF WRL Trq_BrakeReg"
  Demux1/33 -> BusCreator1/33  "PT IF WRL Trq_Supp2WC"
  Demux1/32 -> BusCreator1/32  "PT IF WRL Trq_Drive"
  Demux1/31 -> BusCreator1/31  "PT IF WRL Trq_B2W"
  Demux1/30 -> BusCreator1/30  "PT IF WRL rotv"
  Demux1/29 -> BusCreator1/29  "PT IF WRL rot"
  Demux1/28 -> BusCreator1/28  "PT IF WFR Trq_BrakeReg_max"
  Demux1/27 -> BusCreator1/27  "PT IF WFR Trq_BrakeReg"
  Demux1/26 -> BusCreator1/26  "PT IF WFR Trq_Supp2WC"
  Demux1/25 -> BusCreator1/25  "PT IF WFR Trq_Drive"
  Demux1/24 -> BusCreator1/24  "PT IF WFR Trq_B2W"
  Demux1/23 -> BusCreator1/23  "PT IF WFR rotv"
  Demux1/22 -> BusCreator1/22  "PT IF WFR rot"
  Demux1/21 -> BusCreator1/21  "PT IF WFL Trq_BrakeReg_max"
  Demux1/20 -> BusCreator1/20  "PT IF WFL Trq_BrakeReg"
  Demux1/19 -> BusCreator1/19  "PT IF WFL Trq_Supp2WC"
  Demux1/18 -> BusCreator1/18  "PT IF WFL Trq_Drive"
  Demux1/17 -> BusCreator1/17  "PT IF WFL Trq_B2W"
  Demux1/16 -> BusCreator1/16  "PT IF WFL rotv"
  Demux1/15 -> BusCreator1/15  "PT IF WFL rot"
  Demux1/14 -> BusCreator1/14  "PT IF DL_iDiff_mean"
  Demux1/13 -> BusCreator1/13  "PT IF Trq_Supp2BdyEng y"
  Demux1/12 -> BusCreator1/12  "PT IF Trq_Supp2BdyEng x"
  Demux1/11 -> BusCreator1/11  "PT IF Trq_Supp2Bdy1B z"
  Demux1/10 -> BusCreator1/10  "PT IF Trq_Supp2Bdy1B y"
  Demux1/9 -> BusCreator1/9  "PT IF Trq_Supp2Bdy1B x"
  Demux1/8 -> BusCreator1/8  "PT IF Trq_Supp2Bdy1 z"
  Demux1/7 -> BusCreator1/7  "PT IF Trq_Supp2Bdy1 y"
  Demux1/6 -> BusCreator1/6  "PT IF Trq_Supp2Bdy1 x"
  Demux1/5 -> BusCreator1/5  "PT IF Engine_rotv"
  Demux1/4 -> BusCreator1/4  "PT IF GearNo"
  Demux1/3 -> BusCreator1/3  "PT IF OperationError"
  Demux1/2 -> BusCreator1/2  "PT IF OperationState"
  Demux1/1 -> BusCreator1/1  "PT IF Ignition"
  Sync_In/1 -> PowerTrain/1
  PowerTrain/2 -> Terminator/1
  PowerTrainUpd/1 -> Sync_Out/1
  PowerTrain/1 -> PowerTrainUpd/1  "Sync"
  Vhcl.Wheel.PT/1 -> PowerTrain/2
  Brake.IF.Out/1 -> User RearDriven PowerTrain/2(BrakingTorques)
  SD2232.data/1 -> User RearDriven PowerTrain/4(SD2231.data)
  Car.TrqT2W/1 -> User RearDriven PowerTrain/3(ResistanceTorques)
  VhclCtrl.PT/1 -> User RearDriven PowerTrain/1(VhclCtrl), PowerTrain/3
  User RearDriven PowerTrain/1(PowerTrainOut) -> Demux1/1

== system SD2231_Lab1_2024_PIDController/CarMaker/IPG Vehicle/VehicleSource_BuiltIn ==
  u : Inport
  Compare : RelationalOperator  Operator=~=  OutDataTypeStr=boolean  ZeroCross=off
  Constant : Constant  DisableCoverage=on  Value=const  OutDataTypeStr=Inherit: Inherit via back propagation
  y : Outport  VectorParamsAs1DForOutWhenUnconnected=off
  wires:
  Compare/1 -> y/1
  Constant/1 -> Compare/2
  u/1 -> Compare/1

== system SD2231_Lab1_2024_PIDController/CarMaker/VehicleControl/CreateBus Vhcl.Misc ==
  In1 : Inport
  BusCreator : BusCreator  Inputs=11
  Demux : Demux  Outputs=11
      settings: DisplayOption=none
  Out1 : Outport  VectorParamsAs1DForOutWhenUnconnected=off
  wires:
  Demux/11 -> BusCreator/11  "Vhcl Wind_vel_0 z"
  Demux/10 -> BusCreator/10  "Vhcl Wind_vel_0 y"
  Demux/9 -> BusCreator/9  "Vhcl Wind_vel_0 x"
  Demux/8 -> BusCreator/8  "Vhcl Trq_DL2BdyEng y"
  Demux/7 -> BusCreator/7  "Vhcl Trq_DL2BdyEng x"
  Demux/6 -> BusCreator/6  "Vhcl Trq_DL2Bdy1B z"
  Demux/5 -> BusCreator/5  "Vhcl Trq_DL2Bdy1B y"
  Demux/4 -> BusCreator/4  "Vhcl Trq_DL2Bdy1B x"
  Demux/3 -> BusCreator/3  "Vhcl Trq_DL2Bdy1 z"
  Demux/2 -> BusCreator/2  "Vhcl Trq_DL2Bdy1 y"
  Demux/1 -> BusCreator/1  "Vhcl Trq_DL2Bdy1 x"
  In1/1 -> Demux/1
  BusCreator/1 -> Out1/1

== system SD2231_Lab1_2024_PIDController/CarMaker/VehicleControl/CreateBus Vhcl.Wheel.In ==
  In1 : Inport
  Bus Creator1 : BusCreator  Inputs=12
  Demux1 : Demux  Outputs=12
      settings: DisplayOption=none
  Out1 : Outport  VectorParamsAs1DForOutWhenUnconnected=off
  wires:
  Demux1/12 -> Bus Creator1/12  "Vhcl Wheel RR rotv"
  Demux1/11 -> Bus Creator1/11  "Vhcl Wheel RR Trq_DL2WC"
  Demux1/10 -> Bus Creator1/10  "Vhcl Wheel RR Trq_B2WC"
  Demux1/9 -> Bus Creator1/9  "Vhcl Wheel RL rotv"
  Demux1/8 -> Bus Creator1/8  "Vhcl Wheel RL Trq_DL2WC"
  Demux1/7 -> Bus Creator1/7  "Vhcl Wheel RL Trq_B2WC"
  Demux1/6 -> Bus Creator1/6  "Vhcl Wheel FR rotv"
  Demux1/5 -> Bus Creator1/5  "Vhcl Wheel FR Trq_DL2WC"
  Demux1/4 -> Bus Creator1/4  "Vhcl Wheel FR Trq_B2WC"
  Demux1/3 -> Bus Creator1/3  "Vhcl Wheel FL rotv"
  In1/1 -> Demux1/1
  Bus Creator1/1 -> Out1/1
  Demux1/2 -> Bus Creator1/2  "Vhcl Wheel FL Trq_DL2WC"
  Demux1/1 -> Bus Creator1/1  "Vhcl Wheel FL Trq_B2WC"

== system SD2231_Lab1_2024_PIDController/CarMaker/VehicleControl/CreateBus VhclCtrl ==
  In : Inport
  BusCreator : BusCreator  Inputs=29
  Demux : Demux  Outputs=29
      settings: DisplayOption=none
  Out : Outport  VectorParamsAs1DForOutWhenUnconnected=off
  wires:
  In/1 -> Demux/1
  BusCreator/1 -> Out/1
  Demux/1 -> BusCreator/1  "VhclCtrl SST"
  Demux/2 -> BusCreator/2  "VhclCtrl Key"
  Demux/3 -> BusCreator/3  "VhclCtrl UserSignal0"
  Demux/4 -> BusCreator/4  "VhclCtrl UserSignal1"
  Demux/5 -> BusCreator/5  "VhclCtrl UserSignal2"
  Demux/6 -> BusCreator/6  "VhclCtrl UserSignal3"
  Demux/7 -> BusCreator/7  "VhclCtrl UserSignal4"
  Demux/8 -> BusCreator/8  "VhclCtrl GearNo"
  Demux/9 -> BusCreator/9  "VhclCtrl SelectorCtrl"
  Demux/10 -> BusCreator/10  "VhclCtrl Brake"
  Demux/11 -> BusCreator/11  "VhclCtrl BrakePark"
  Demux/12 -> BusCreator/12  "VhclCtrl Clutch"
  Demux/13 -> BusCreator/13  "VhclCtrl Gas"
  Demux/14 -> BusCreator/14  "VhclCtrl Steering Ang"
  Demux/15 -> BusCreator/15  "VhclCtrl Steering AngVel"
  Demux/16 -> BusCreator/16  "VhclCtrl Steering AngAcc"
  Demux/17 -> BusCreator/17  "VhclCtrl Steering Trq"
  Demux/18 -> BusCreator/18  "VhclCtrl Lights LowBeam"
  Demux/19 -> BusCreator/19  "VhclCtrl Lights HighBeam"
  Demux/20 -> BusCreator/20  "VhclCtrl Lights Daytime"
  Demux/21 -> BusCreator/21  "VhclCtrl Lights ParkL"
  Demux/22 -> BusCreator/22  "VhclCtrl Lights ParkR"
  Demux/23 -> BusCreator/23  "VhclCtrl Lights IndL"
  Demux/24 -> BusCreator/24  "VhclCtrl Lights IndR"
  Demux/25 -> BusCreator/25  "VhclCtrl Lights FogFrontL"
  Demux/26 -> BusCreator/26  "VhclCtrl Lights FogFrontR"
  Demux/27 -> BusCreator/27  "VhclCtrl Lights FogRear"
  Demux/28 -> BusCreator/28  "VhclCtrl Lights Brake"
  Demux/29 -> BusCreator/29  "VhclCtrl Lights Reverse"

== system SD2231_Lab1_2024_PIDController/CarMaker/VehicleControl/CreateBus VhclCtrl.PT ==
  In1 : Inport
  BusCreator1 : BusCreator  Inputs=12
  Demux1 : Demux  Outputs=12
      settings: DisplayOption=none
  Out1 : Outport  VectorParamsAs1DForOutWhenUnconnected=off
  wires:
  Demux1/12 -> BusCreator1/12  "VhclCtrl Brake"
  Demux1/11 -> BusCreator1/11  "VhclCtrl Gas"
  Demux1/10 -> BusCreator1/10  "VhclCtrl Clutch"
  Demux1/9 -> BusCreator1/9  "VhclCtrl SelectorCtrl"
  Demux1/8 -> BusCreator1/8  "VhclCtrl GearNo"
  Demux1/7 -> BusCreator1/7  "VhclCtrl UserSignal4"
  Demux1/6 -> BusCreator1/6  "VhclCtrl UserSignal3"
  Demux1/5 -> BusCreator1/5  "VhclCtrl UserSignal2"
  Demux1/4 -> BusCreator1/4  "VhclCtrl UserSignal1"
  Demux1/3 -> BusCreator1/3  "VhclCtrl UserSignal0"
  Demux1/2 -> BusCreator1/2  "VhclCtrl Key"
  Demux1/1 -> BusCreator1/1  "VhclCtrl SST"
  In1/1 -> Demux1/1
  BusCreator1/1 -> Out1/1

== system SD2231_Lab1_2024_PIDController/CarMaker/VehicleControl/CreateBus VhclCtrl.Steering ==
  In1 : Inport
  Bus Creator : BusCreator  Inputs=5
  Demux : Demux  Outputs=5
      settings: DisplayOption=none
  Out1 : Outport  VectorParamsAs1DForOutWhenUnconnected=off
  wires:
  In1/1 -> Demux/1
  Bus Creator/1 -> Out1/1
  Demux/1 -> Bus Creator/1  "VhclCtrl Steering Ang"
  Demux/5 -> Bus Creator/5  "VhclCtrl Steering SteerByTrq"
  Demux/3 -> Bus Creator/3  "VhclCtrl Steering AngAcc"
  Demux/2 -> Bus Creator/2  "VhclCtrl Steering AngVel"
  Demux/4 -> Bus Creator/4  "VhclCtrl Steering Trq"

== system SD2231_Lab1_2024_PIDController/CarMaker/Your ABS Controller/P Controller ==
  <FL Braking Slip> : Inport
  <RL Braking Slip> : Inport  Port=2
  <Brake pedal> : Inport  Port=3
  Vehicle_Velocity : Inport  Port=4
  P_Front_Breaking : Subsystem
  P_Rear_Breaking : Subsystem
  Sum : Sum  Inputs=|-+
  Sum1 : Sum  Inputs=+-|
  Switch : Switch  Criteria=u2 > Threshold  Threshold=2.5  SaturateOnIntegerOverflow=off  InputSameDT=off
  Switch1 : Switch  Criteria=u2 > Threshold  Threshold=0.05  SaturateOnIntegerOverflow=off  InputSameDT=off
  Switch2 : Switch  Criteria=u2 > Threshold  Threshold=2.5  SaturateOnIntegerOverflow=off  InputSameDT=off
  Switch3 : Switch  Criteria=u2 > Threshold  Threshold=0.05  SaturateOnIntegerOverflow=off  InputSameDT=off
  Front_Braking : Outport
  Rear_Braking : Outport  Port=2
  wires:
  <FL Braking Slip>/1 -> P_Front_Breaking/1(In1), Switch1/2
  P_Front_Breaking/1(Out1) -> Sum/1
  <Brake pedal>/1 -> Switch3/3, Switch2/3, Switch1/3, Switch/3, Sum/2, Sum1/1
  <RL Braking Slip>/1 -> Switch3/2, P_Rear_Breaking/1(In1)
  Sum/1 -> Switch1/1
  Switch1/1 -> Switch/1
  Switch/1 -> Front_Braking/1
  Vehicle_Velocity/1 -> Switch/2, Switch2/2
  Switch3/1 -> Switch2/1
  Switch2/1 -> Rear_Braking/1
  Sum1/1 -> Switch3/1
  P_Rear_Breaking/1(Out1) -> Sum1/2

== system SD2231_Lab1_2024_PIDController/CarMaker/Your ABS Controller/PD Controller ==
  <FL Braking Slip> : Inport
  <RL Braking Slip> : Inport  Port=2
  <Brake pedal> : Inport  Port=3
  Vehicle_Velocity : Inport  Port=4
  PD_Front_Breaking : Subsystem
  PD_Rear_Breaking : Subsystem
  Sum : Sum  Inputs=|-+
  Sum1 : Sum  Inputs=+-|
  Switch : Switch  Criteria=u2 > Threshold  Threshold=2.5  SaturateOnIntegerOverflow=off  InputSameDT=off
  Switch1 : Switch  Criteria=u2 > Threshold  Threshold=0.05  SaturateOnIntegerOverflow=off  InputSameDT=off
  Switch2 : Switch  Criteria=u2 > Threshold  Threshold=2.5  SaturateOnIntegerOverflow=off  InputSameDT=off
  Switch3 : Switch  Criteria=u2 > Threshold  Threshold=0.05  SaturateOnIntegerOverflow=off  InputSameDT=off
  Front_Braking : Outport
  Rear_Braking : Outport  Port=2
  wires:
  <FL Braking Slip>/1 -> PD_Front_Breaking/1(In1), Switch1/2
  PD_Front_Breaking/1(Out1) -> Sum/1
  <Brake pedal>/1 -> Switch3/3, Switch2/3, Switch1/3, Switch/3, Sum/2, Sum1/1
  <RL Braking Slip>/1 -> PD_Rear_Breaking/1(In1), Switch3/2
  Sum/1 -> Switch1/1
  Switch1/1 -> Switch/1
  Switch/1 -> Front_Braking/1
  Vehicle_Velocity/1 -> Switch/2, Switch2/2
  Switch3/1 -> Switch2/1
  Switch2/1 -> Rear_Braking/1
  Sum1/1 -> Switch3/1
  PD_Rear_Breaking/1(Out1) -> Sum1/2

== system SD2231_Lab1_2024_PIDController/CarMaker/Your ABS Controller/PI Controller ==
  <FL Braking Slip> : Inport
  <RL Braking Slip> : Inport  Port=2
  <Brake pedal> : Inport  Port=3
  Vehicle_Velocity : Inport  Port=4
  PI_Front_Breaking : Subsystem
  PI_Rear_Breaking : Subsystem
  Sum : Sum  Inputs=|-+
  Sum1 : Sum  Inputs=+-|
  Switch : Switch  Criteria=u2 > Threshold  Threshold=2.5  SaturateOnIntegerOverflow=off  InputSameDT=off
  Switch1 : Switch  Criteria=u2 > Threshold  Threshold=0.05  SaturateOnIntegerOverflow=off  InputSameDT=off
  Switch2 : Switch  Criteria=u2 > Threshold  Threshold=2.5  SaturateOnIntegerOverflow=off  InputSameDT=off
  Switch3 : Switch  Criteria=u2 > Threshold  Threshold=0.05  SaturateOnIntegerOverflow=off  InputSameDT=off
  Front_Braking : Outport
  Rear_Braking : Outport  Port=2
  wires:
  <FL Braking Slip>/1 -> PI_Front_Breaking/1(In1), Switch1/2
  PI_Front_Breaking/1(Out1) -> Sum/1
  <Brake pedal>/1 -> Switch3/3, Switch2/3, Switch1/3, Switch/3, Sum/2, Sum1/1
  <RL Braking Slip>/1 -> PI_Rear_Breaking/1(In1), Switch3/2
  Sum/1 -> Switch1/1
  Switch1/1 -> Switch/1
  Switch/1 -> Front_Braking/1
  Vehicle_Velocity/1 -> Switch/2, Switch2/2
  Switch3/1 -> Switch2/1
  Switch2/1 -> Rear_Braking/1
  Sum1/1 -> Switch3/1
  PI_Rear_Breaking/1(Out1) -> Sum1/2

== system SD2231_Lab1_2024_PIDController/CarMaker/Your ABS Controller/PID Controller ==
  <FL Braking Slip> : Inport
  <RL Braking Slip> : Inport  Port=2
  <Brake pedal> : Inport  Port=3
  Vehicle_Velocity : Inport  Port=4
  PID_Front_Breaking : Subsystem
  PID_Rear_Breaking : Subsystem
  Sum : Sum  Inputs=|-+
  Sum1 : Sum  Inputs=+-|
  Switch : Switch  Criteria=u2 > Threshold  Threshold=2.5  SaturateOnIntegerOverflow=off  InputSameDT=off
  Switch1 : Switch  Criteria=u2 > Threshold  Threshold=0.05  SaturateOnIntegerOverflow=off  InputSameDT=off
  Switch2 : Switch  Criteria=u2 > Threshold  Threshold=2.5  SaturateOnIntegerOverflow=off  InputSameDT=off
  Switch3 : Switch  Criteria=u2 > Threshold  Threshold=0.05  SaturateOnIntegerOverflow=off  InputSameDT=off
  Front_Braking : Outport
  Rear_Braking : Outport  Port=2
  wires:
  <FL Braking Slip>/1 -> PID_Front_Breaking/1(In1), Switch1/2
  PID_Front_Breaking/1(Out1) -> Sum/1
  <Brake pedal>/1 -> Switch3/3, Switch2/3, Switch1/3, Switch/3, Sum/2, Sum1/1
  <RL Braking Slip>/1 -> PID_Rear_Breaking/1(In1), Switch3/2
  Sum/1 -> Switch1/1
  Switch1/1 -> Switch/1
  Switch/1 -> Front_Braking/1
  Vehicle_Velocity/1 -> Switch/2, Switch2/2
  Switch3/1 -> Switch2/1
  Switch2/1 -> Rear_Braking/1
  Sum1/1 -> Switch3/1
  PID_Rear_Breaking/1(Out1) -> Sum1/2

== system SD2231_Lab1_2024_PIDController/CarMaker/IPG Vehicle/Brake/CreateBus Vhcl.Wheel.PT ==
  In : Inport
  BusCreator1 : BusCreator  Inputs=20
  Demux1 : Demux  Outputs=20
      settings: DisplayOption=none
  Out : Outport  VectorParamsAs1DForOutWhenUnconnected=off
  wires:
  Demux1/20 -> BusCreator1/20  "Vhcl Trq_DriveSrc_trg d3"
  Demux1/19 -> BusCreator1/19  "Vhcl Trq_DriveSrc_trg d2"
  Demux1/18 -> BusCreator1/18  "Vhcl Trq_DriveSrc_trg d1"
  Demux1/17 -> BusCreator1/17  "Vhcl Trq_DriveSrc_trg d0"
  Demux1/16 -> BusCreator1/16  "Vhcl Wheel RR WhlBearing"
  Demux1/15 -> BusCreator1/15  "Vhcl Wheel RR Trq_T2W"
  Demux1/14 -> BusCreator1/14  "Vhcl Wheel RR Trq_BrakeReg_trg"
  Demux1/13 -> BusCreator1/13  "Vhcl Wheel RR Trq_Brake"
  Demux1/12 -> BusCreator1/12  "Vhcl Wheel RL WhlBearing"
  Demux1/11 -> BusCreator1/11  "Vhcl Wheel RL Trq_T2W"
  Demux1/10 -> BusCreator1/10  "Vhcl Wheel RL Trq_BrakeReg_trg"
  Demux1/9 -> BusCreator1/9  "Vhcl Wheel RL Trq_Brake"
  Demux1/8 -> BusCreator1/8  "Vhcl Wheel FR WhlBearing"
  Demux1/7 -> BusCreator1/7  "Vhcl Wheel FR Trq_T2W"
  Demux1/6 -> BusCreator1/6  "Vhcl Wheel FR Trq_BrakeReg_trg"
  Demux1/5 -> BusCreator1/5  "Vhcl Wheel FR Trq_Brake"
  Demux1/4 -> BusCreator1/4  "Vhcl Wheel FL WhlBearing"
  Demux1/3 -> BusCreator1/3  "Vhcl Wheel FL Trq_T2W"
  Demux1/2 -> BusCreator1/2  "Vhcl Wheel FL Trq_BrakeReg_trg"
  Demux1/1 -> BusCreator1/1  "Vhcl Wheel FL Trq_Brake"
  BusCreator1/1 -> Out/1
  In/1 -> Demux1/1

== system SD2231_Lab1_2024_PIDController/CarMaker/IPG Vehicle/Brake/UserDefinedBrakingSystem ==
  note: Please note: Influence of DrivMan.Handbrake on the braking
      | torques (Brake IF Trq_XX signals) is ignored in this example.
  SD2231.Data : Inport
  Bus Creator2 : BusCreator  Inputs=16
  Bus Selector : BusSelector  OutputSignals=FLBrakeAdjust,FRBrakeAdjust,RLBrakeAdjust,RRBrakeAdjust
  Constant : Constant  Value=0
  NOTSET : Constant  Value=-99999
  Subsystem : Subsystem
  Subsystem1 : Subsystem
  Subsystem2 : Subsystem
  Subsystem3 : Subsystem
  Brake.IF.Out : Outport  VectorParamsAs1DForOutWhenUnconnected=off
  wires:
  SD2231.Data/1 -> Bus Selector/1
  Bus Creator2/1 -> Brake.IF.Out/1
  Constant/1 -> Bus Creator2/10, Bus Creator2/5, Bus Creator2/6, Bus Creator2/7, Bus Creator2/8, Bus Creator2/9, Bus Creator2/11, Bus Creator2/12
  NOTSET/1 -> Bus Creator2/13, Bus Creator2/14, Bus Creator2/15, Bus Creator2/16
  Subsystem/1(FL brake force) -> Bus Creator2/1
  Bus Selector/1 -> Subsystem/1(FLBrakeAdjust)  "<FLBrakeAdjust>"
  Subsystem1/1(FR brake force) -> Bus Creator2/2
  Subsystem2/1(RL brake force) -> Bus Creator2/3
  Subsystem3/1(RR brake force) -> Bus Creator2/4
  Bus Selector/2 -> Subsystem1/1(FRBrakeAdjust)  "<FRBrakeAdjust>"
  Bus Selector/3 -> Subsystem2/1(RLBrakeAdjust)  "<RLBrakeAdjust>"
  Bus Selector/4 -> Subsystem3/1(RRBrakeAdjust)  "<RRBrakeAdjust>"
